simulink model "Sleep_Mech"  (Simulink 6.4)
settings: Solver=ode23tb  StartTime=0.0  StopTime=3600*(24*1+10)  RelTol=1e-3
values from neighbouring files (symbols this model uses):
  Circadian_Period = 24    [Respiratory_IC.m]    (also in State_UA_Khoo_IC.m)
  fc = 0.4/60    (= 0.00666666666667)    [Respiratory_IC.m]    (also in State_UA_Khoo_IC.m)
  gc = 0.008/60    (= 0.000133333333333)    [Respiratory_IC.m]    (also in State_UA_Khoo_IC.m)
  rc = 0.2/60    (= 0.00333333333333)    [Respiratory_IC.m]    (also in State_UA_Khoo_IC.m)
  Sleep = 0    [Respiratory_IC.m]    (also in State_UA_Khoo_IC.m)
  SWAo = 0.007    [Respiratory_IC.m]    (also in State_UA_Khoo_IC.m)
libraries: simulink x2
settings Model: LastModifiedBy=CLM
settings ConfigSet: SimulationMode=accelerator
settings OptimizationCC: BlockReduction=off  BooleanDataType=off

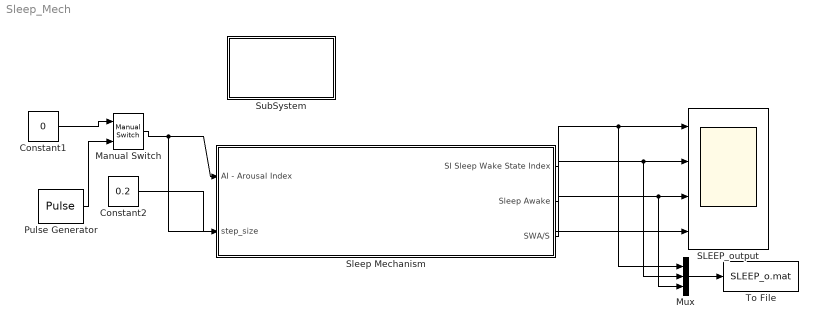
== system Sleep_Mech ==
  Constant1 : Constant  Value=0  OutDataType=sfix(16)  ConRadixGroup=Use specified scaling  OutScaling=2^0  SampleTime=inf  FramePeriod=inf
  Constant2 : Constant  Value=0.2  OutDataType=sfix(16)  ConRadixGroup=Use specified scaling  OutScaling=2^0  SampleTime=inf  FramePeriod=inf
  Manual Switch : simulink/Signal Routing/Manual Switch  SystemSampleTime=-1  sw=1  action=0
  Mux : Mux  Inputs=3
  Pulse Generator : DiscretePulseGenerator  PulseType=Time based  Period=90  PulseWidth=(30/90)*100  PhaseDelay=2000
  SLEEP_output : Scope  NumInputPorts=4
      settings: YMin=-0.05~-0.05~-0.05~-0.05  YMax=1.05~1.05~1.05~1.05
  Sleep Mechanism : Subsystem
  SubSystem : Subsystem
      settings: OpenFcn=State_UA_Khoo_IC
      mask Display: disp('"double click here"\n to load \nState_UA_Khoo \ninitial values');
  To File : ToFile  Filename=SLEEP_o.mat  MatrixName=SI_SleepAwake_SWAS
  wires:
  Sleep Mechanism/1(SI Sleep Wake State Index) -> SLEEP_output/1, Mux/1
  Sleep Mechanism/3(SWA/S) -> SLEEP_output/3, Mux/3
  Sleep Mechanism/2(Sleep Awake) -> SLEEP_output/2, Mux/2
  Mux/1 -> To File/1
  Constant1/1 -> Manual Switch/1
  Manual Switch/1 -> Sleep Mechanism/1(AI - Arousal Index), SLEEP_output/4
  Pulse Generator/1 -> Manual Switch/2
  Constant2/1 -> Sleep Mechanism/2(step_size)

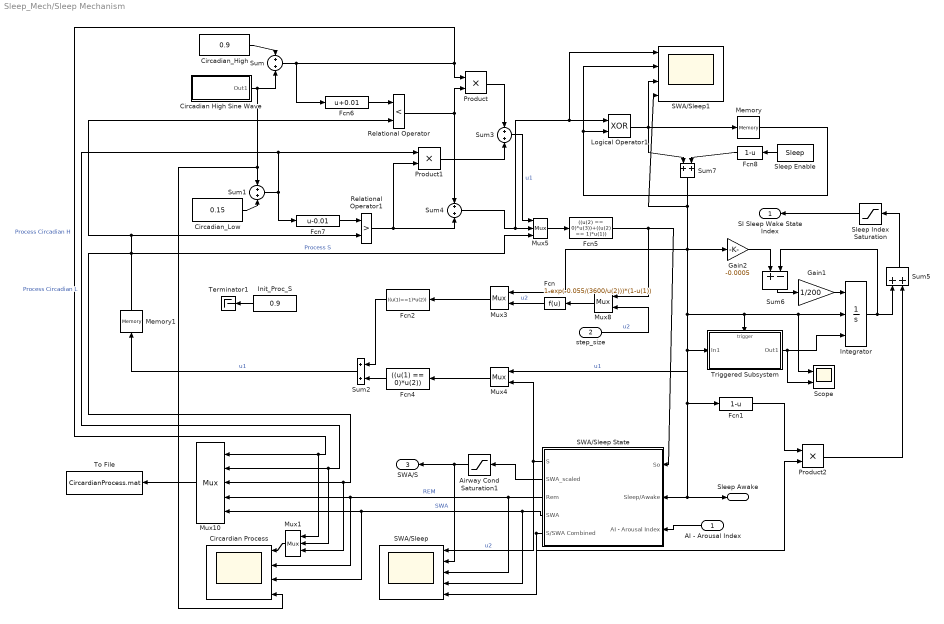
== system Sleep_Mech/Sleep Mechanism ==
  AI - Arousal Index : Inport  Orientation=left
  step_size : Inport  Port=2
  Airway Cond Saturation1 : Saturate  Orientation=left  UpperLimit=1  LowerLimit=0
  Circadian High Sine Wave : Subsystem
  Circadian_High : Constant  Value=0.9  OutDataType=sfix(16)  ConRadixGroup=Use specified scaling  OutScaling=2^0  SampleTime=inf  FramePeriod=inf
  Circadian_Low : Constant  Value=0.15  OutDataType=sfix(16)  ConRadixGroup=Use specified scaling  OutScaling=2^0  SampleTime=inf  FramePeriod=inf
  Circardian Process : Scope  NumInputPorts=4
      settings: YMin=0.005~-0.05~0.01~-0.15  YMax=1.05~1.05~0.95~0.15
  Fcn : Fcn  Orientation=left  Expr=1-exp(-0.055/(3600/u(2)))*(1-u(1))
  Fcn1 : Fcn  Expr=1-u
  Fcn2 : Fcn  Orientation=left  Expr=((u(1)==1)*u(2))
  Fcn4 : Fcn  Orientation=left  Expr=((u(1) == 0)*u(2))
  Fcn5 : Fcn  Expr=((u(2) == 0)*u(3))+((u(2) == 1)*u(1))
  Fcn6 : Fcn  Expr=u+0.01
  Fcn7 : Fcn  Expr=u-0.01
  Fcn8 : Fcn  Orientation=left  Expr=1-u
  Gain1 : Gain  Gain=1/200  SaturateOnIntegerOverflow=on
  Gain2 : Gain  Gain=-0.0005  SaturateOnIntegerOverflow=on
  Init_Proc_S : Constant  Orientation=left  Value=0.9  OutDataType=sfix(16)  ConRadixGroup=Use specified scaling  OutScaling=2^0  SampleTime=inf  FramePeriod=inf
  Integrator : Integrator  ExternalReset=rising  InitialConditionSource=external  InitialCondition=1
  Logical Operator1 : Logic  Operator=XOR
  Memory : Memory  X0=1  InheritSampleTime=on
  Memory1 : Memory  Orientation=up  X0=1  InheritSampleTime=on
  Mux1 : Mux  Orientation=left  Inputs=3
  Mux10 : Mux  Orientation=left  Inputs=5
  Mux3 : Mux  Orientation=left  Inputs=2
  Mux4 : Mux  Orientation=left  Inputs=2
  Mux5 : Mux  Inputs=3
  Mux8 : Mux  Orientation=left  Inputs=2
  Product : Product  SaturateOnIntegerOverflow=on  InputSameDT=on
  Product1 : Product  SaturateOnIntegerOverflow=on  InputSameDT=on
  Product2 : Product  SaturateOnIntegerOverflow=on  InputSameDT=on
  Relational Operator : RelationalOperator  Operator=<  InputSameDT=on
  Relational Operator1 : RelationalOperator  Operator=>  InputSameDT=on
  SWA/Sleep : Scope  NumInputPorts=5
      settings: YMin=0~0~0~0~0  YMax=1~1~1~1~1  SaveName=ScopeData2
  SWA/Sleep State : Subsystem  Orientation=left
  SWA/Sleep1 : Scope  NumInputPorts=4
      settings: YMin=-0.05~-0.05~-0.05~-0.05  YMax=1.05~1.05~1.05~1.05  SaveName=ScopeData3
  Scope : Scope  NumInputPorts=2
      settings: YMin=-0.05~-0.05  YMax=1.05~1.05  SaveName=ScopeData5  MaxDataPoints=500
  Sleep Enable : Constant  Orientation=left  Value=Sleep  OutDataType=sfix(16)  ConRadixGroup=Use specified scaling  OutScaling=2^0  SampleTime=inf  FramePeriod=inf
  Sleep Index Saturation : Saturate  Orientation=left  UpperLimit=1  LowerLimit=0
  Sum{,1,3..4} (4 alike) : Sum  SaturateOnIntegerOverflow=on  InputSameDT=on
  Sum2 : Sum  Orientation=left  SaturateOnIntegerOverflow=on  InputSameDT=on
  Sum5 : Sum  Orientation=up  SaturateOnIntegerOverflow=on  InputSameDT=on
  Sum6 : Sum  Orientation=down  Inputs=+-  SaturateOnIntegerOverflow=on  InputSameDT=on
  Sum7 : Sum  Orientation=down  SaturateOnIntegerOverflow=on  InputSameDT=on
  Terminator1 : Terminator
  To File : ToFile  Orientation=left  Filename=CircardianProcess.mat  MatrixName=H_L_CircardianLow_RBM_SWA
  Triggered Subsystem : Subsystem  TreatAsAtomicUnit=on
  SI Sleep Wake State Index : Outport  Orientation=left
  Sleep Awake : Outport  Port=2
  SWA/S : Outport  Orientation=left  Port=3
  wires:
  AI - Arousal Index/1 -> SWA/Sleep State/3(AI - Arousal Index)
  Circadian_High/1 -> Sum/1
  Circadian High Sine Wave/1(Out1) -> Sum/2, Sum1/1, Circardian Process/4
  Circadian_Low/1 -> Sum1/2
  Sum/1 -> Fcn6/1, Product/1, Mux10/1, Mux1/1  "Process Circadian H"
  Sum1/1 -> Fcn7/1, Product1/1, Mux10/2, Mux1/2  "Process Circadian L"
  Memory/1 -> Logical Operator1/2, SWA/Sleep1/2
  Logical Operator1/1 -> Memory/1, Sum7/1, SWA/Sleep1/3
  Relational Operator/1 -> Product/2, Sum4/1
  Relational Operator1/1 -> Sum4/2, Product1/2
  Product/1 -> Sum3/1
  Product1/1 -> Sum3/2
  Sum3/1 -> Mux5/1  "u1"
  Fcn2/1 -> Sum2/1
  Fcn4/1 -> Sum2/2
  Sum2/1 -> Memory1/1  "u1"
  Fcn/1 -> Mux3/2  "u2"
  SWA/Sleep State/1(S) -> Mux4/2, SWA/Sleep/1  "u2"
  Sum4/1 -> Mux5/2, Logical Operator1/1, SWA/Sleep1/1
  Mux5/1 -> Fcn5/1
  Mux3/1 -> Fcn2/1
  Mux4/1 -> Fcn4/1
  Fcn5/1 -> SWA/Sleep State/1(So), Mux8/1
  Fcn6/1 -> Relational Operator/1
  Fcn7/1 -> Relational Operator1/1
  Mux8/1 -> Fcn/1
  step_size/1 -> Mux8/2  "u2"
  SWA/Sleep State/2(SWA_scaled) -> Airway Cond Saturation1/1
  Airway Cond Saturation1/1 -> SWA/S/1, SWA/Sleep/2
  Mux10/1 -> To File/1
  SWA/Sleep State/3(Rem) -> Mux10/4, Circardian Process/2, SWA/Sleep/3  "REM"
  SWA/Sleep State/4(SWA) -> Mux10/5, Circardian Process/3, SWA/Sleep/4  "SWA"
  SWA/Sleep State/5(S/SWA Combined) -> Product2/2, SWA/Sleep/5
  Fcn1/1 -> Product2/1
  Sum5/1 -> Sleep Index Saturation/1
  Product2/1 -> Sum5/2
  Sleep Index Saturation/1 -> SI Sleep Wake State Index/1
  Sum7/1 -> Gain2/1, Mux3/1, Triggered Subsystem/Trigger, Integrator/2, Scope/1, Fcn1/1, Mux4/1, Sleep Awake/1, SWA/Sleep State/2(Sleep/Awake), Triggered Subsystem/1(In1), SWA/Sleep1/4  "u1"
  Integrator/1 -> Sum5/1, Sum6/2
  Triggered Subsystem/1(Out1) -> Integrator/3, Scope/2
  Gain2/1 -> Sum6/1
  Sum6/1 -> Gain1/1
  Gain1/1 -> Integrator/1
  Sleep Enable/1 -> Fcn8/1
  Fcn8/1 -> Sum7/2
  Init_Proc_S/1 -> Terminator1/1
  Memory1/1 -> Mux5/3, Mux10/3, Mux1/3, Relational Operator/2, Relational Operator1/2  "Process S"
  Mux1/1 -> Circardian Process/1

== system Sleep_Mech/SubSystem ==

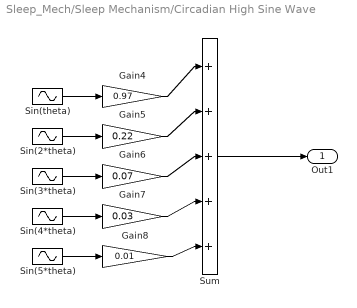
== system Sleep_Mech/Sleep Mechanism/Circadian High Sine Wave ==
  Gain4 : Gain  Gain=0.97  SaturateOnIntegerOverflow=on
  Gain5 : Gain  Gain=0.22  SaturateOnIntegerOverflow=on
  Gain6 : Gain  Gain=0.07  SaturateOnIntegerOverflow=on
  Gain7 : Gain  Gain=0.03  SaturateOnIntegerOverflow=on
  Gain8 : Gain  Gain=0.01  SaturateOnIntegerOverflow=on
  Sin(2*theta) : Sin  Amplitude=0.12  Frequency=(2*2*pi)/(Circadian_Period*3600)  Phase=3.2358  SampleTime=0
  Sin(3*theta) : Sin  Amplitude=0.12  Frequency=(3*2*pi)/(Circadian_Period*3600)  Phase=3.2358  SampleTime=0
  Sin(4*theta) : Sin  Amplitude=0.12  Frequency=(4*2*pi)/(Circadian_Period*3600)  Phase=3.2358  SampleTime=0
  Sin(5*theta) : Sin  Amplitude=0.12  Frequency=(5*2*pi)/(Circadian_Period*3600)  Phase=3.2358  SampleTime=0
  Sin(theta) : Sin  Amplitude=0.12  Frequency=(2*pi)/(Circadian_Period*3600)  Phase=3.2358  SampleTime=0
  Sum : Sum  Inputs=|+++++  SaturateOnIntegerOverflow=on  InputSameDT=on
  Out1 : Outport
  wires:
  Sin(theta)/1 -> Gain4/1
  Gain4/1 -> Sum/1
  Sin(2*theta)/1 -> Gain5/1
  Gain5/1 -> Sum/2
  Sin(3*theta)/1 -> Gain6/1
  Gain6/1 -> Sum/3
  Sin(4*theta)/1 -> Gain7/1
  Gain7/1 -> Sum/4
  Sin(5*theta)/1 -> Gain8/1
  Gain8/1 -> Sum/5
  Sum/1 -> Out1/1

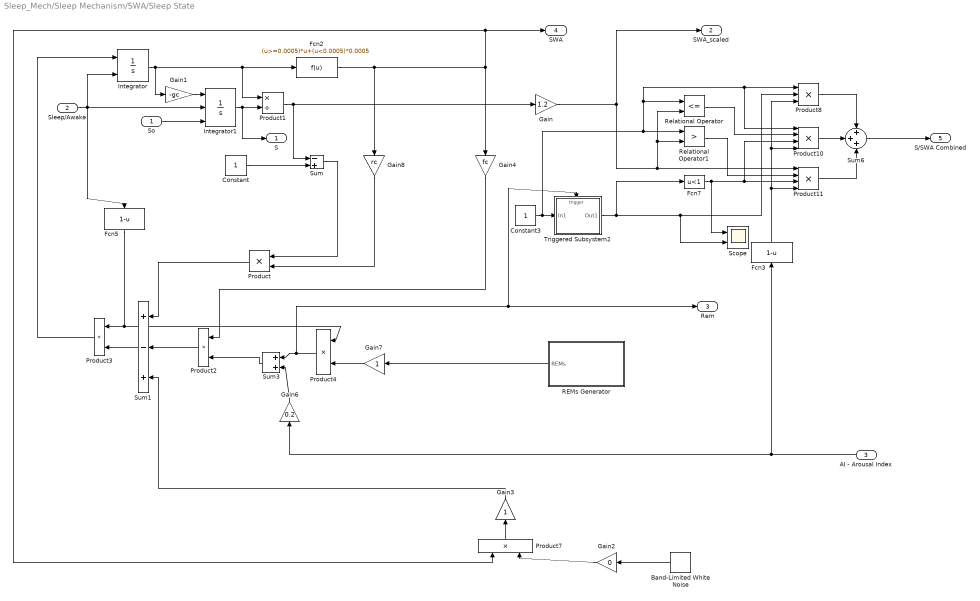
== system Sleep_Mech/Sleep Mechanism/SWA/Sleep State ==
  So : Inport
  Sleep/Awake : Inport  Port=2
  AI - Arousal Index : Inport  Orientation=left  Port=3
  Band-Limited White Noise : simulink/Sources/Band-Limited White Noise  Orientation=left  SystemSampleTime=-1  Cov=[0.1]  Ts=0.1  seed=[23341]
  Constant : Constant  Value=1  OutDataType=sfix(16)  ConRadixGroup=Use specified scaling  OutScaling=2^0  SampleTime=inf  FramePeriod=inf
  Constant3 : Constant  Value=1  OutDataType=sfix(16)  ConRadixGroup=Use specified scaling  OutScaling=2^0  SampleTime=inf  FramePeriod=inf
  Fcn2 : Fcn  Expr=(u>=0.0005)*u+(u<0.0005)*0.0005
  Fcn3 : Fcn  Orientation=up  Expr=1-u
  Fcn5 : Fcn  Orientation=down  Expr=1-u
  Fcn7 : Fcn  Expr=u<1
  Gain : Gain  Gain=1.2
  Gain1 : Gain  Gain=-gc  SaturateOnIntegerOverflow=on
  Gain2 : Gain  Orientation=left  Gain=0  SaturateOnIntegerOverflow=on
  Gain3 : Gain  Orientation=up  SaturateOnIntegerOverflow=on
  Gain4 : Gain  Orientation=down  Gain=fc  SaturateOnIntegerOverflow=on
  Gain6 : Gain  Orientation=up  Gain=0.2  SaturateOnIntegerOverflow=on
  Gain7 : Gain  Orientation=left  SaturateOnIntegerOverflow=on
  Gain8 : Gain  Orientation=down  Gain=rc  SaturateOnIntegerOverflow=on
  Integrator : Integrator  ExternalReset=either  InitialCondition=SWAo  LimitOutput=on  UpperSaturationLimit=1  LowerSaturationLimit=0
  Integrator1 : Integrator  ExternalReset=falling  InitialConditionSource=external  InitialCondition=0.8  LimitOutput=on
  Product : Product  Orientation=left  SaturateOnIntegerOverflow=on  InputSameDT=on
  Product1 : Product  Inputs=*/  SaturateOnIntegerOverflow=on  InputSameDT=on
  Product10 : Product  Inputs=4  SaturateOnIntegerOverflow=on  InputSameDT=on
  Product11 : Product  Inputs=4  SaturateOnIntegerOverflow=on  InputSameDT=on
  Product2 : Product  Orientation=left  SaturateOnIntegerOverflow=on  InputSameDT=on
  Product3 : Product  Orientation=left  SaturateOnIntegerOverflow=on  InputSameDT=on
  Product4 : Product  Orientation=left  Inputs=**  SaturateOnIntegerOverflow=on  InputSameDT=on
  Product7 : Product  Orientation=up  SaturateOnIntegerOverflow=on  InputSameDT=on
  Product8 : Product  Inputs=3  SaturateOnIntegerOverflow=on  InputSameDT=on
  REMs Generator : Subsystem  Orientation=left
  Relational Operator : RelationalOperator  Operator=<=  InputSameDT=on
  Relational Operator1 : RelationalOperator  Operator=>  InputSameDT=on
  Scope : Scope  NumInputPorts=2
      settings: YMin=-0.05~-0.05  YMax=1.05~1.05  SaveName=ScopeData4  MaxDataPoints=500
  Sum : Sum  Inputs=-+  SaturateOnIntegerOverflow=on  InputSameDT=on
  Sum1 : Sum  Orientation=left  Inputs=+-+  SaturateOnIntegerOverflow=on  InputSameDT=on
  Sum3 : Sum  Orientation=left  SaturateOnIntegerOverflow=on  InputSameDT=on
  Sum6 : Sum  Inputs=+++  SaturateOnIntegerOverflow=on  InputSameDT=on
  Triggered Subsystem2 : Subsystem  TreatAsAtomicUnit=on
  S : Outport
  SWA_scaled : Outport  Port=2
  Rem : Outport  Port=3
  SWA : Outport  Port=4
  S/SWA Combined : Outport  Port=5
  wires:
  Relational Operator1/1 -> Product11/2
  Fcn7/1 -> Product11/3, Product10/3, Scope/1
  Product10/1 -> Sum6/2
  Product11/1 -> Sum6/3
  Relational Operator/1 -> Product10/2
  Sum6/1 -> S/SWA Combined/1
  Product8/1 -> Sum6/1
  Constant3/1 -> Triggered Subsystem2/1(In1), Relational Operator1/1, Relational Operator/1, Product8/1, Product10/1
  Gain2/1 -> Product7/2
  Product7/1 -> Gain3/1
  Gain6/1 -> Sum3/2
  AI - Arousal Index/1 -> Gain6/1, Fcn3/1
  Sum3/1 -> Product2/2
  Constant/1 -> Sum/2
  Product1/1 -> Sum/1, Gain/1
  Gain1/1 -> Integrator1/1
  Integrator/1 -> Product1/1, Fcn2/1, Gain1/1
  Sum/1 -> Product/1
  Product/1 -> Sum1/1
  Product2/1 -> Sum1/2
  Gain3/1 -> Sum1/3
  Integrator1/1 -> Product1/2, S/1
  Sleep/Awake/1 -> Integrator1/2, Fcn5/1, Integrator/2
  So/1 -> Integrator1/3
  Fcn2/1 -> Gain4/1, Product7/1, SWA/1, Gain8/1
  Gain/1 -> Relational Operator1/2, Relational Operator/2, Product11/1, SWA_scaled/1
  Gain4/1 -> Product2/1
  Gain8/1 -> Product/2
  Sum1/1 -> Product3/2
  Product3/1 -> Integrator/1
  Fcn5/1 -> Product3/1, Product4/1
  REMs Generator/1(REMs) -> Gain7/1
  Fcn3/1 -> Product8/3, Product10/4, Product11/4
  Product4/1 -> Sum3/1, Rem/1, Triggered Subsystem2/Trigger
  Band-Limited White Noise/1 -> Gain2/1
  Gain7/1 -> Product4/2
  Triggered Subsystem2/1(Out1) -> Fcn7/1, Product8/2, Scope/2

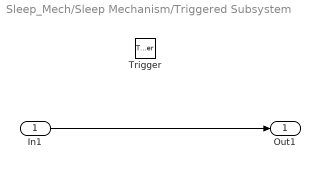
== system Sleep_Mech/Sleep Mechanism/Triggered Subsystem ==
  In1 : Inport
  Trigger : TriggerPort
  Out1 : Outport
  wires:
  In1/1 -> Out1/1

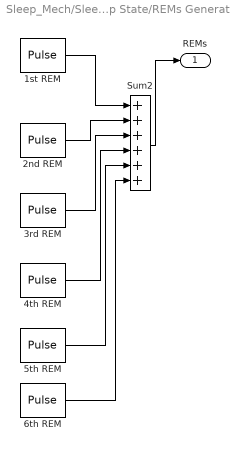
== system Sleep_Mech/Sleep Mechanism/SWA/Sleep State/REMs Generator ==
  1st REM : DiscretePulseGenerator  PulseType=Time based  Period=Circadian_Period*3600  PulseWidth=(100-85) *1.8 /Circadian_Period  PhaseDelay=3600*1.8*0.85+5
  2nd REM : DiscretePulseGenerator  PulseType=Time based  Period=Circadian_Period*3600  PulseWidth=(100-85) *1.8 /Circadian_Period  PhaseDelay=3600*1.8*(1+0.85)+5
  3rd REM : DiscretePulseGenerator  PulseType=Time based  Period=Circadian_Period*3600  PulseWidth=(100-85) *1.8 /Circadian_Period  PhaseDelay=3600*1.8*(2+0.85)+5
  4th REM : DiscretePulseGenerator  PulseType=Time based  Period=Circadian_Period*3600  PulseWidth=(100-85) *1.8 /Circadian_Period  PhaseDelay=3600*1.8*(3+0.85)+5
  5th REM : DiscretePulseGenerator  PulseType=Time based  Period=Circadian_Period*3600  PulseWidth=(100-85) *1.8 /Circadian_Period  PhaseDelay=3600*1.8*(4+0.85)+5
  6th REM : DiscretePulseGenerator  PulseType=Time based  Period=Circadian_Period*3600  PulseWidth=(100-85) *1.8 /Circadian_Period  PhaseDelay=3600*1.8*(5+0.85)+5
  Sum2 : Sum  Inputs=++++++  SaturateOnIntegerOverflow=on  InputSameDT=on
  REMs : Outport
  wires:
  Sum2/1 -> REMs/1
  1st REM/1 -> Sum2/1
  2nd REM/1 -> Sum2/2
  3rd REM/1 -> Sum2/3
  4th REM/1 -> Sum2/4
  5th REM/1 -> Sum2/5
  6th REM/1 -> Sum2/6

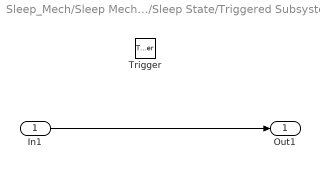
== system Sleep_Mech/Sleep Mechanism/SWA/Sleep State/Triggered Subsystem2 ==
  In1 : Inport
  Trigger : TriggerPort
  Out1 : Outport
  wires:
  In1/1 -> Out1/1
